simulink model "Crazyflie_NoLinealModel_EB_2020b"  (R2020b)
settings: Solver=FixedStepAuto  StartTime=0.0  StopTime=30  FixedStep=0.001  RelTol=1e-3
undefined symbols (not defined in the file): DiscIntNeverNeededParam, Dphi_s, Dphi_T, Dpsi_s, Dtheta_s, fm, MCO, Phi_s, Phi_T, phi_theta_limit, quad, Theta_s, U_q, V_q, we, X_q, XY_delta, XY_T, xyv_lim, Y_q, Yaw_delta, Yaw_q, Yaw_T, Z_delta, Z_s, Z_T
libraries: pid_lib x6, simulink x4
settings Model: Creator=Rafael  LastModifiedBy=FranciscoJose
settings DataIOCC: LimitDataPoints=on  SaveFormat=Array  SignalLoggingSaveFormat=ModelDataLogs  ReturnWorkspaceOutputs=off
settings OptimizationCC: ExpressionDepthLimit=2147483647  LifeSpan=inf
settings DebuggingCC: UnderspecifiedInitializationDetection=Classic  MergeDetectMultiDrivingBlocksExec=none  SolverPrmCheckMsg=warning  FcnCallInpInsideContextMsg=warning  AllowSymbolicDim=off  StateNameClashWarn=warning  SFUnexpectedBacktrackingDiag=warning  SFNoUnconditionalDefaultTransitionDiag=warning  SFExecutionAtInitializationDiag=none  ArithmeticOperatorsInVariantConditions=warning
settings HardwareCC: ProdBitPerPointer=32  ProdBitPerSizeT=32  ProdBitPerPtrDiffT=32  ProdLargestAtomicFloat=None  ProdIntDivRoundTo=Undefined  ProdEndianess=Unspecified  ProdWordSize=32  ProdHWDeviceType=32-bit Generic
settings ModelReferenceCC: PropagateSignalLabelsOutOfModel=off
settings SFSimCC: SimUseLocalCustomCode=off  CustomCodeUndefinedFunction=UseInterfaceOnly
settings RTWCC: RTWUseLocalCustomCode=off
settings CodeAppCC: StateflowObjectComments=on
settings GRTTargetCC: TargetLangStandard=C89/C90 (ANSI)
settings ConfigComp: CovMetricSettings=dw  CovSaveCumulativeToWorkspaceVar=on  CovSaveSingleToWorkspaceVar=on  CovExternalEMLEnable=off
settings SimscapeCC: SimscapeNormalizeSystem=off
settings ConfigurationSet: Description=SimMechanics 2G

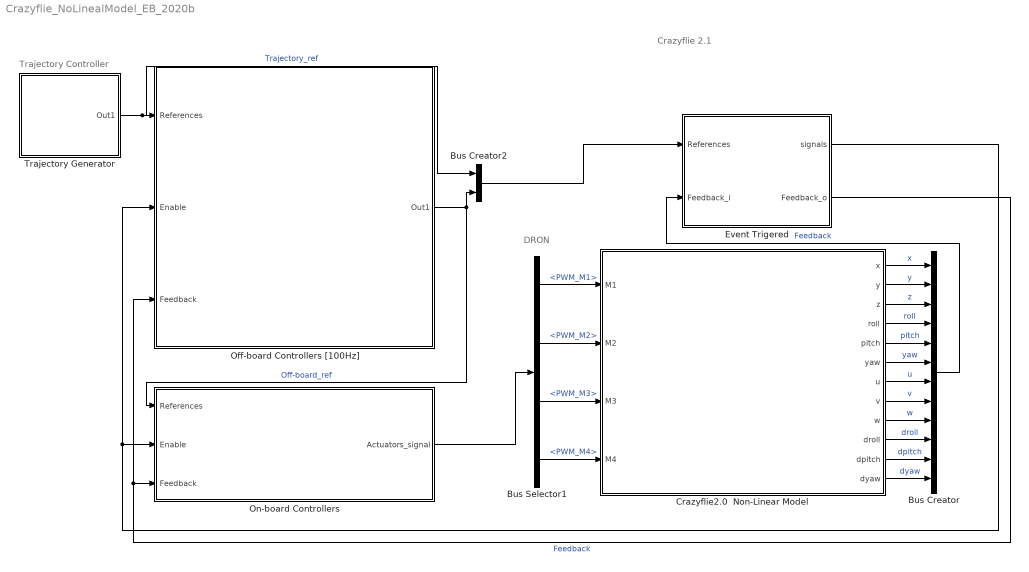
== system Crazyflie_NoLinealModel_EB_2020b ==
  note: DRON
  note: Trajectory Controller
  note: Crazyflie 2.1
  Bus Creator : BusCreator  Inputs=12
  Bus Creator2 : BusCreator  Inputs=2
  Bus Selector1 : BusSelector  OutputSignals=PWM_M1,PWM_M2,PWM_M3,PWM_M4
  Crazyflie2.0  Non-Linear Model : Subsystem
      mask Display: image('crazyflie_icon.png')
  Event Trigered : Subsystem
  Off-board Controllers [100Hz] : Subsystem
  On-board Controllers : Subsystem
  Trajectory Generator : Subsystem
  wires:
  Crazyflie2.0  Non-Linear Model/11(dpitch) -> Bus Creator/11  "dpitch"
  Crazyflie2.0  Non-Linear Model/3(z) -> Bus Creator/3  "z"
  Crazyflie2.0  Non-Linear Model/12(dyaw) -> Bus Creator/12  "dyaw"
  Crazyflie2.0  Non-Linear Model/4(roll) -> Bus Creator/4  "roll"
  Crazyflie2.0  Non-Linear Model/5(pitch) -> Bus Creator/5  "pitch"
  Crazyflie2.0  Non-Linear Model/6(yaw) -> Bus Creator/6  "yaw"
  Crazyflie2.0  Non-Linear Model/1(x) -> Bus Creator/1  "x"
  Crazyflie2.0  Non-Linear Model/2(y) -> Bus Creator/2  "y"
  Crazyflie2.0  Non-Linear Model/7(u) -> Bus Creator/7  "u"
  Crazyflie2.0  Non-Linear Model/8(v) -> Bus Creator/8  "v"
  Crazyflie2.0  Non-Linear Model/9(w) -> Bus Creator/9  "w"
  Crazyflie2.0  Non-Linear Model/10(droll) -> Bus Creator/10  "droll"
  Event Trigered/2(Feedback_o) -> Off-board Controllers [100Hz]/3(Feedback), On-board Controllers/3(Feedback)  "Feedback"
  Bus Selector1/1 -> Crazyflie2.0  Non-Linear Model/1(M1)  "<PWM_M1>"
  Bus Selector1/2 -> Crazyflie2.0  Non-Linear Model/2(M2)  "<PWM_M2>"
  Bus Selector1/3 -> Crazyflie2.0  Non-Linear Model/3(M3)  "<PWM_M3>"
  Bus Selector1/4 -> Crazyflie2.0  Non-Linear Model/4(M4)  "<PWM_M4>"
  Trajectory Generator/1(Out1) -> Bus Creator2/1, Off-board Controllers [100Hz]/1(References)  "Trajectory_ref"
  Bus Creator2/1 -> Event Trigered/1(References)
  Bus Creator/1 -> Event Trigered/2(Feedback_i)  "Feedback"
  Event Trigered/1(signals) -> Off-board Controllers [100Hz]/2(Enable), On-board Controllers/2(Enable)
  On-board Controllers/1(Actuators_signal) -> Bus Selector1/1
  Off-board Controllers [100Hz]/1(Out1) -> On-board Controllers/1(References), Bus Creator2/2  "Off-board_ref"

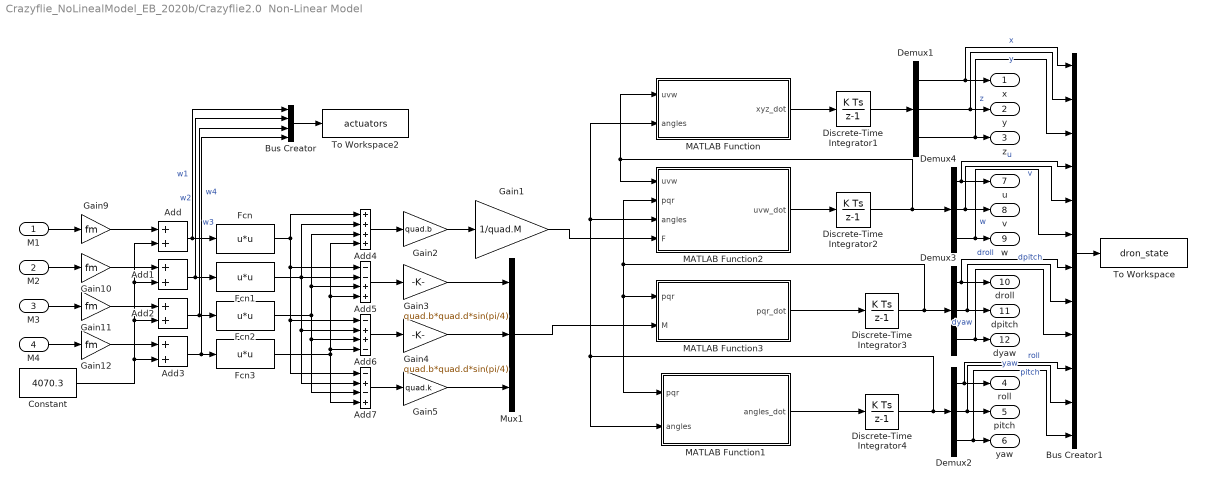
== system Crazyflie_NoLinealModel_EB_2020b/Crazyflie2.0  Non-Linear Model ==
  M1 : Inport
  M2 : Inport  Port=2
  M3 : Inport  Port=3
  M4 : Inport  Port=4
  Add{,1..3} (4 alike) : Sum
  Add4 : Sum  Inputs=++++
  Add5 : Sum  Inputs=--++
  Add6 : Sum  Inputs=-++-
  Add7 : Sum  Inputs=-+-+
  Bus Creator : BusCreator  Inputs=4
  Bus Creator1 : BusCreator  Inputs=12
  Constant : Constant  Value=4070.3
  Demux{1..4} (4 alike) : Demux  Outputs=3
  Discrete-Time Integrator{1..4} (4 alike) : DiscreteIntegrator  SampleTime=0.001  ICPrevOutput=DiscIntNeverNeededParam  ICPrevScaledInput=DiscIntNeverNeededParam
  Fcn{,1..3} (4 alike) : Fcn  Expr=u*u
  Gain1 : Gain  Gain=1/quad.M
  Gain{9..12} (4 alike) : Gain  Gain=fm
  Gain2 : Gain  Gain=quad.b
  Gain3 : Gain  Gain=quad.b*quad.d*sin(pi/4)
  Gain4 : Gain  Gain=quad.b*quad.d*sin(pi/4)
  Gain5 : Gain  Gain=quad.k
  MATLAB Function : MATLAB Function  TreatAsAtomicUnit=on
  MATLAB Function1 : MATLAB Function  TreatAsAtomicUnit=on
  MATLAB Function2 : MATLAB Function  TreatAsAtomicUnit=on
  MATLAB Function3 : MATLAB Function  TreatAsAtomicUnit=on
  Mux1 : Mux  Inputs=3
  To Workspace : ToWorkspace  VariableName=dron_state  SaveFormat=Timeseries  SampleTime=-1
  To Workspace2 : ToWorkspace  VariableName=actuators  SaveFormat=Timeseries  SampleTime=-1
  x : Outport
  y : Outport  Port=2
  z : Outport  Port=3
  roll : Outport  Port=4
  pitch : Outport  Port=5
  yaw : Outport  Port=6
  u : Outport  Port=7
  v : Outport  Port=8
  w : Outport  Port=9
  droll : Outport  Port=10
  dpitch : Outport  Port=11
  dyaw : Outport  Port=12
  wires:
  Demux1/1 -> Bus Creator1/1, x/1  "x"
  Demux1/2 -> Bus Creator1/2, y/1  "y"
  Demux2/1 -> Bus Creator1/10, roll/1  "roll"
  Demux2/2 -> Bus Creator1/11, pitch/1  "pitch"
  Demux2/3 -> Bus Creator1/12, yaw/1  "yaw"
  Demux4/1 -> Bus Creator1/4, u/1  "u"
  Demux4/2 -> Bus Creator1/5, v/1  "v"
  Demux4/3 -> Bus Creator1/6, w/1  "w"
  Demux3/1 -> Bus Creator1/7, droll/1  "droll"
  Demux3/2 -> Bus Creator1/8, dpitch/1  "dpitch"
  Demux3/3 -> Bus Creator1/9, dyaw/1  "dyaw"
  M1/1 -> Gain9/1
  M2/1 -> Gain10/1
  M3/1 -> Gain11/1
  M4/1 -> Gain12/1
  Add/1 -> Bus Creator/1, Fcn/1  "w1"
  Add1/1 -> Bus Creator/2, Fcn1/1  "w2"
  Add2/1 -> Bus Creator/3, Fcn2/1  "w3"
  Add3/1 -> Bus Creator/4, Fcn3/1  "w4"
  Gain9/1 -> Add/1
  Gain10/1 -> Add1/1
  Gain11/1 -> Add2/1
  Gain12/1 -> Add3/1
  Constant/1 -> Add3/2, Add/2, Add1/2, Add2/2
  Discrete-Time Integrator3/1 -> Demux3/1, MATLAB Function2/2(pqr), MATLAB Function1/1(pqr), MATLAB Function3/1(pqr)
  Discrete-Time Integrator2/1 -> MATLAB Function2/1(uvw), MATLAB Function/1(uvw), Demux4/1
  MATLAB Function3/1(pqr_dot) -> Discrete-Time Integrator3/1
  MATLAB Function1/1(angles_dot) -> Discrete-Time Integrator4/1
  Mux1/1 -> MATLAB Function3/2(M)
  Discrete-Time Integrator4/1 -> Demux2/1, MATLAB Function1/2(angles), MATLAB Function/2(angles), MATLAB Function2/3(angles)
  Discrete-Time Integrator1/1 -> Demux1/1
  MATLAB Function/1(xyz_dot) -> Discrete-Time Integrator1/1
  Gain4/1 -> Mux1/2
  Add6/1 -> Gain4/1
  Gain5/1 -> Mux1/3
  Gain3/1 -> Mux1/1
  Gain1/1 -> MATLAB Function2/4(F)
  Fcn2/1 -> Add4/3, Add5/3, Add7/3, Add6/3
  Add7/1 -> Gain5/1
  Fcn/1 -> Add4/1, Add7/1, Add6/1, Add5/1
  Add5/1 -> Gain3/1
  Fcn3/1 -> Add4/4, Add5/4, Add6/4, Add7/4
  Fcn1/1 -> Add4/2, Add7/2, Add6/2, Add5/2
  Gain2/1 -> Gain1/1
  Add4/1 -> Gain2/1
  MATLAB Function2/1(uvw_dot) -> Discrete-Time Integrator2/1
  Bus Creator/1 -> To Workspace2/1
  Bus Creator1/1 -> To Workspace/1
  Demux1/3 -> Bus Creator1/3, z/1  "z"

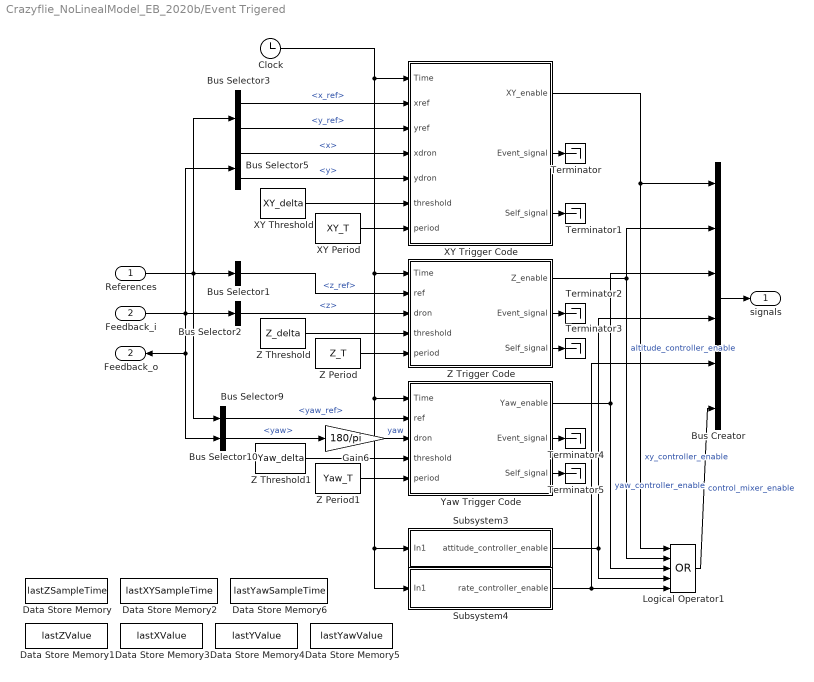
== system Crazyflie_NoLinealModel_EB_2020b/Event Trigered ==
  References : Inport
  Feedback_i : Inport  Port=2
  Bus Creator : BusCreator  Inputs=6
  Bus Selector1 : BusSelector  OutputSignals=Trajectory_ref.z_ref
  Bus Selector10 : BusSelector  OutputSignals=yaw
  Bus Selector2 : BusSelector  OutputSignals=z
  Bus Selector3 : BusSelector  OutputSignals=Trajectory_ref.x_ref,Trajectory_ref.y_ref
  Bus Selector5 : BusSelector  OutputSignals=x,y
  Bus Selector9 : BusSelector  OutputSignals=Trajectory_ref.yaw_ref
  Clock : Clock
  Data Store Memory : DataStoreMemory  DataStoreName=lastZSampleTime  InitialValue=0.0  ShowAdditionalParam=off  OutDataTypeStr=double
  Data Store Memory1 : DataStoreMemory  DataStoreName=lastZValue  InitialValue=0.0  ShowAdditionalParam=off  OutDataTypeStr=double
  Data Store Memory2 : DataStoreMemory  DataStoreName=lastXYSampleTime  InitialValue=0.0  ShowAdditionalParam=off  OutDataTypeStr=double
  Data Store Memory3 : DataStoreMemory  DataStoreName=lastXValue  InitialValue=0.0  ShowAdditionalParam=off  OutDataTypeStr=double
  Data Store Memory4 : DataStoreMemory  DataStoreName=lastYValue  InitialValue=0.0  ShowAdditionalParam=off  OutDataTypeStr=double
  Data Store Memory5 : DataStoreMemory  DataStoreName=lastYawValue  InitialValue=0.0  ShowAdditionalParam=off  OutDataTypeStr=double
  Data Store Memory6 : DataStoreMemory  DataStoreName=lastYawSampleTime  InitialValue=0.0  ShowAdditionalParam=off  OutDataTypeStr=double
  Gain6 : Gain  Gain=180/pi
  Logical Operator1 : Logic  Operator=OR  Inputs=5  AllPortsSameDT=off  OutDataTypeStr=boolean
  Subsystem3 : Subsystem
  Subsystem4 : Subsystem
  Terminator{,1..5} (6 alike) : Terminator
  XY Period : Constant  Value=XY_T
  XY Threshold : Constant  Value=XY_delta
  XY Trigger Code : MATLAB Function  TreatAsAtomicUnit=on
  Yaw Trigger Code : MATLAB Function  TreatAsAtomicUnit=on
  Z Period : Constant  Value=Z_T
  Z Period1 : Constant  Value=Yaw_T
  Z Threshold : Constant  Value=Z_delta
  Z Threshold1 : Constant  Value=Yaw_delta
  Z Trigger Code : MATLAB Function  TreatAsAtomicUnit=on
  signals : Outport
  Feedback_o : Outport  Port=2
  wires:
  References/1 -> Bus Selector9/1, Bus Selector1/1, Bus Selector3/1
  Bus Selector9/1 -> Yaw Trigger Code/2(ref)  "<yaw_ref>"
  Bus Selector10/1 -> Gain6/1  "<yaw>"
  Bus Creator/1 -> signals/1
  Gain6/1 -> Yaw Trigger Code/3(dron)  "yaw"
  Logical Operator1/1 -> Bus Creator/6  "control_mixer_enable"
  Z Trigger Code/1(Z_enable) -> Logical Operator1/2, Bus Creator/2  "altitude_controller_enable"
  XY Trigger Code/1(XY_enable) -> Logical Operator1/1, Bus Creator/1  "xy_controller_enable"
  Yaw Trigger Code/1(Yaw_enable) -> Logical Operator1/3, Bus Creator/3  "yaw_controller_enable"
  Subsystem3/1(attitude_controller_enable) -> Bus Creator/4, Logical Operator1/4
  Clock/1 -> Subsystem4/1(In1), Subsystem3/1(In1), Yaw Trigger Code/1(Time), Z Trigger Code/1(Time), XY Trigger Code/1(Time)
  Subsystem4/1(rate_controller_enable) -> Logical Operator1/5, Bus Creator/5
  Z Threshold/1 -> Z Trigger Code/4(threshold)
  Z Period/1 -> Z Trigger Code/5(period)
  Bus Selector1/1 -> Z Trigger Code/2(ref)  "<z_ref>"
  Bus Selector2/1 -> Z Trigger Code/3(dron)  "<z>"
  Bus Selector3/1 -> XY Trigger Code/2(xref)  "<x_ref>"
  Bus Selector3/2 -> XY Trigger Code/3(yref)  "<y_ref>"
  Feedback_i/1 -> Bus Selector2/1, Bus Selector5/1, Bus Selector10/1, Feedback_o/1
  Bus Selector5/1 -> XY Trigger Code/4(xdron)  "<x>"
  Bus Selector5/2 -> XY Trigger Code/5(ydron)  "<y>"
  XY Threshold/1 -> XY Trigger Code/6(threshold)
  XY Period/1 -> XY Trigger Code/7(period)
  XY Trigger Code/2(Event_signal) -> Terminator/1
  XY Trigger Code/3(Self_signal) -> Terminator1/1
  Z Threshold1/1 -> Yaw Trigger Code/4(threshold)
  Z Period1/1 -> Yaw Trigger Code/5(period)
  Yaw Trigger Code/2(Event_signal) -> Terminator4/1
  Yaw Trigger Code/3(Self_signal) -> Terminator5/1
  Z Trigger Code/2(Event_signal) -> Terminator2/1
  Z Trigger Code/3(Self_signal) -> Terminator3/1

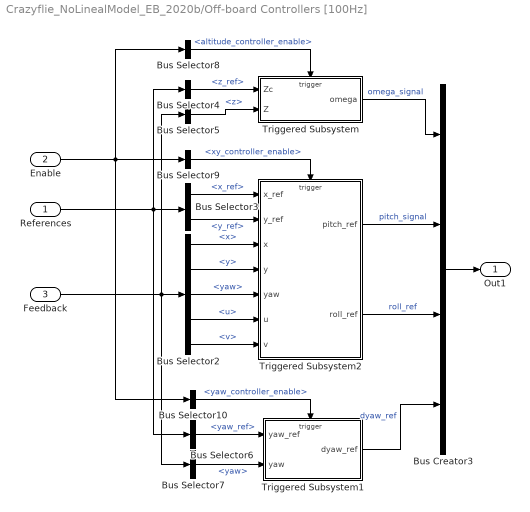
== system Crazyflie_NoLinealModel_EB_2020b/Off-board Controllers [100Hz] ==
  References : Inport
  Enable : Inport  Port=2
  Feedback : Inport  Port=3
  Bus Creator3 : BusCreator  Inputs=4
  Bus Selector10 : BusSelector  OutputSignals=yaw_controller_enable
  Bus Selector2 : BusSelector  OutputSignals=x,y,yaw,u,v
  Bus Selector3 : BusSelector  OutputSignals=x_ref,y_ref
  Bus Selector4 : BusSelector  OutputSignals=z_ref
  Bus Selector5 : BusSelector  OutputSignals=z
  Bus Selector6 : BusSelector  OutputSignals=yaw_ref
  Bus Selector7 : BusSelector  OutputSignals=yaw
  Bus Selector8 : BusSelector  OutputSignals=altitude_controller_enable
  Bus Selector9 : BusSelector  OutputSignals=xy_controller_enable
  Triggered Subsystem : Subsystem  TreatAsAtomicUnit=on
  Triggered Subsystem1 : Subsystem  TreatAsAtomicUnit=on
  Triggered Subsystem2 : Subsystem  TreatAsAtomicUnit=on
  Out1 : Outport
  wires:
  Bus Selector2/3 -> Triggered Subsystem2/5(yaw)  "<yaw>"
  Bus Selector6/1 -> Triggered Subsystem1/1(yaw_ref)  "<yaw_ref>"
  Bus Selector2/5 -> Triggered Subsystem2/7(v)  "<v>"
  References/1 -> Bus Selector4/1, Bus Selector3/1, Bus Selector6/1
  Triggered Subsystem2/1(pitch_ref) -> Bus Creator3/2  "pitch_signal"
  Enable/1 -> Bus Selector10/1, Bus Selector8/1, Bus Selector9/1
  Feedback/1 -> Bus Selector7/1, Bus Selector5/1, Bus Selector2/1
  Bus Selector2/1 -> Triggered Subsystem2/3(x)  "<x>"
  Bus Selector7/1 -> Triggered Subsystem1/2(yaw)  "<yaw>"
  Bus Selector2/4 -> Triggered Subsystem2/6(u)  "<u>"
  Bus Selector4/1 -> Triggered Subsystem/1(Zc)  "<z_ref>"
  Bus Selector3/1 -> Triggered Subsystem2/1(x_ref)  "<x_ref>"
  Bus Selector3/2 -> Triggered Subsystem2/2(y_ref)  "<y_ref>"
  Bus Selector2/2 -> Triggered Subsystem2/4(y)  "<y>"
  Triggered Subsystem2/2(roll_ref) -> Bus Creator3/3  "roll_ref"
  Bus Selector5/1 -> Triggered Subsystem/2(Z)  "<z>"
  Triggered Subsystem1/1(dyaw_ref) -> Bus Creator3/4  "dyaw_ref"
  Bus Selector9/1 -> Triggered Subsystem2/Trigger  "<xy_controller_enable>"
  Bus Selector10/1 -> Triggered Subsystem1/Trigger  "<yaw_controller_enable>"
  Bus Selector8/1 -> Triggered Subsystem/Trigger  "<altitude_controller_enable>"
  Bus Creator3/1 -> Out1/1
  Triggered Subsystem/1(omega) -> Bus Creator3/1  "omega_signal"

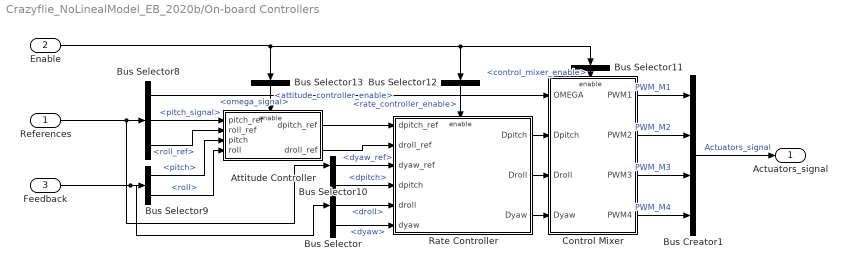
== system Crazyflie_NoLinealModel_EB_2020b/On-board Controllers ==
  References : Inport
  Enable : Inport  Port=2
  Feedback : Inport  Port=3
  Attitude Controller : Subsystem  TreatAsAtomicUnit=on
  Bus Creator1 : BusCreator  Inputs=4
  Bus Selector : BusSelector  OutputSignals=dpitch,droll,dyaw
  Bus Selector10 : BusSelector  OutputSignals=dyaw_ref
  Bus Selector11 : BusSelector  OutputSignals=control_mixer_enable
  Bus Selector12 : BusSelector  OutputSignals=rate_controller_enable
  Bus Selector13 : BusSelector  OutputSignals=attitude_controller_enable
  Bus Selector8 : BusSelector  OutputSignals=omega_signal,pitch_signal,roll_ref
  Bus Selector9 : BusSelector  OutputSignals=pitch,roll
  Control Mixer : Subsystem  TreatAsAtomicUnit=on
  Rate Controller : Subsystem  TreatAsAtomicUnit=on
  Actuators_signal : Outport
  wires:
  Bus Creator1/1 -> Actuators_signal/1  "Actuators_signal"
  Bus Selector/2 -> Rate Controller/5(droll)  "<droll>"
  Control Mixer/3(PWM3) -> Bus Creator1/3  "PWM_M3"
  Rate Controller/3(Dyaw) -> Control Mixer/4(Dyaw)
  Enable/1 -> Bus Selector11/1, Bus Selector12/1, Bus Selector13/1
  Bus Selector8/2 -> Attitude Controller/1(pitch_ref)  "<pitch_signal>"
  Bus Selector8/3 -> Attitude Controller/2(roll_ref)  "<roll_ref>"
  References/1 -> Bus Selector8/1, Bus Selector10/1
  Bus Selector12/1 -> Rate Controller/Enable  "<rate_controller_enable>"
  Attitude Controller/2(droll_ref) -> Rate Controller/2(droll_ref)
  Bus Selector10/1 -> Rate Controller/3(dyaw_ref)  "<dyaw_ref>"
  Bus Selector/1 -> Rate Controller/4(dpitch)  "<dpitch>"
  Bus Selector/3 -> Rate Controller/6(dyaw)  "<dyaw>"
  Feedback/1 -> Bus Selector/1, Bus Selector9/1
  Control Mixer/4(PWM4) -> Bus Creator1/4  "PWM_M4"
  Attitude Controller/1(dpitch_ref) -> Rate Controller/1(dpitch_ref)
  Rate Controller/1(Dpitch) -> Control Mixer/2(Dpitch)
  Rate Controller/2(Droll) -> Control Mixer/3(Droll)
  Bus Selector8/1 -> Control Mixer/1(OMEGA)  "<omega_signal>"
  Control Mixer/2(PWM2) -> Bus Creator1/2  "PWM_M2"
  Control Mixer/1(PWM1) -> Bus Creator1/1  "PWM_M1"
  Bus Selector9/2 -> Attitude Controller/4(roll)  "<roll>"
  Bus Selector9/1 -> Attitude Controller/3(pitch)  "<pitch>"
  Bus Selector11/1 -> Control Mixer/Enable  "<control_mixer_enable>"
  Bus Selector13/1 -> Attitude Controller/Enable  "<attitude_controller_enable>"

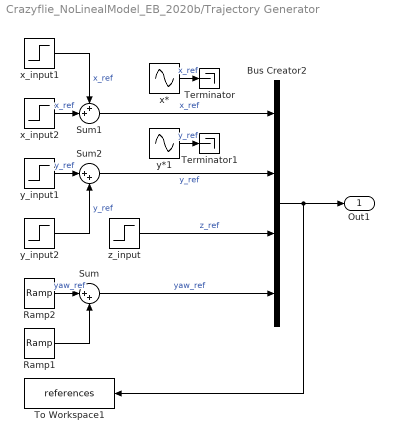
== system Crazyflie_NoLinealModel_EB_2020b/Trajectory Generator ==
  Bus Creator2 : BusCreator  Inputs=4
  Ramp1 : simulink/Sources/Ramp  slope=-pi/3  start=10  InitialOutput=0
  Ramp2 : simulink/Sources/Ramp  slope=pi/3  start=0  InitialOutput=0
  Sum : Sum  Inputs=|++
  Sum1 : Sum  Inputs=++|
  Sum2 : Sum  Inputs=|++
  Terminator : Terminator
  Terminator1 : Terminator
  To Workspace1 : ToWorkspace  VariableName=references  SaveFormat=Timeseries  SampleTime=-1
  x* : Sin  Amplitude=0.8  Frequency=2*pi*0.085  Phase=0-0.1  SampleTime=0
  x_input1 : Step  Time=6  SampleTime=0
  x_input2 : Step  Time=18  After=-1  SampleTime=0
  y*1 : Sin  Amplitude=0.8  Frequency=2*pi*0.085  Phase=pi/2-0.1  SampleTime=0
  y_input1 : Step  Time=12  SampleTime=0
  y_input2 : Step  Time=24  After=-1  SampleTime=0
  z_input : Step  Time=0  SampleTime=0
  Out1 : Outport
  wires:
  z_input/1 -> Bus Creator2/3  "z_ref"
  Sum1/1 -> Bus Creator2/1  "x_ref"
  Ramp1/1 -> Sum/2
  Sum2/1 -> Bus Creator2/2  "y_ref"
  Bus Creator2/1 -> To Workspace1/1, Out1/1
  Sum/1 -> Bus Creator2/4  "yaw_ref"
  Ramp2/1 -> Sum/1  "yaw_ref"
  x_input2/1 -> Sum1/2  "x_ref"
  x_input1/1 -> Sum1/1  "x_ref"
  y_input1/1 -> Sum2/1  "y_ref"
  y_input2/1 -> Sum2/2  "y_ref"
  x*/1 -> Terminator/1  "x_ref"
  y*1/1 -> Terminator1/1  "y_ref"

== system Crazyflie_NoLinealModel_EB_2020b/Event Trigered/Subsystem3 ==
  In1 : Inport
  Compare To Constant4 : simulink/Logic and Bit Operations/Compare To Constant  relop=>=  const=Phi_T  OutDataTypeStr=boolean
  If Action Subsystem4 : Subsystem  TreatAsAtomicUnit=on
  Memory4 : Memory
  Sum8 : Sum  Inputs=|+-
  attitude_controller_enable : Outport
  wires:
  In1/1 -> Sum8/1, If Action Subsystem4/1(In2)
  If Action Subsystem4/1(Out2) -> Memory4/1
  Compare To Constant4/1 -> attitude_controller_enable/1, If Action Subsystem4/Enable  "attitude_controller_enable"
  Memory4/1 -> Sum8/2
  Sum8/1 -> Compare To Constant4/1

== system Crazyflie_NoLinealModel_EB_2020b/Event Trigered/Subsystem4 ==
  In1 : Inport
  Compare To Constant4 : simulink/Logic and Bit Operations/Compare To Constant  relop=>=  const=Dphi_T  OutDataTypeStr=boolean
  If Action Subsystem4 : Subsystem  TreatAsAtomicUnit=on
  Memory4 : Memory
  Sum8 : Sum  Inputs=|+-
  rate_controller_enable : Outport
  wires:
  In1/1 -> Sum8/1, If Action Subsystem4/1(In2)
  Sum8/1 -> Compare To Constant4/1
  If Action Subsystem4/1(Out2) -> Memory4/1
  Compare To Constant4/1 -> rate_controller_enable/1, If Action Subsystem4/Enable  "rate_controller_enable"
  Memory4/1 -> Sum8/2

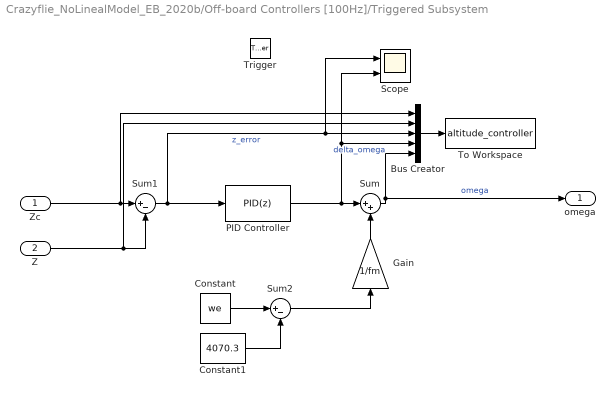
== system Crazyflie_NoLinealModel_EB_2020b/Off-board Controllers [100Hz]/Triggered Subsystem ==
  Zc : Inport
  Z : Inport  Port=2
  Trigger : TriggerPort  VariantControl=Variant
  Bus Creator : BusCreator  Inputs=5
  Constant : Constant  Value=we
  Constant1 : Constant  Value=4070.3
  Gain : Gain  Gain=1/fm
  PID Controller : pid_lib/PID Controller  Controller=PID  Form=Parallel  TimeDomain=Discrete-time  UseExternalTs=off  SampleTime=-1  IntegratorMethod=Forward Euler  FilterMethod=Forward Euler  ControllerParametersSource=internal  P=Z_s(1)  I=Z_s(2)  D=Z_s(3)  UseFilter=on  N=100  TunerSelectOption=Transfer Function Based (PID Tuner App)  InitialConditionSource=internal  InitialConditionForIntegrator=0  InitialConditionForFilter=0  DifferentiatorICPrevScaledInput=0  ExternalReset=none  TrackingMode=off  Kt=1  LimitOutput=on  SatLimitsSource=internal  UpperSaturationLimit=15000  LowerSaturationLimit=-20000  LinearizeAsGain=on  AntiWindupMode=none  Kb=1/sqrt(0.75)  POutMin=[]  POutMax=[]  IOutMin=[]  IOutMax=[]  DOutMin=[]  DOutMax=[]  NOutMin=[]  NOutMax=[]  SumOutMin=[]  SumOutMax=[]  SaturationOutMin=[]  SaturationOutMax=[]  PParamMin=[]  PParamMax=[]  IParamMin=[]  IParamMax=[]  DParamMin=[]  DParamMax=[]  NParamMin=[]  NParamMax=[]  KbParamMin=[]  KbParamMax=[]  KtParamMin=[]  KtParamMax=[]  KbOutMin=[]  KbOutMax=[]  KtOutMin=[]  KtOutMax=[]  IntegratorOutMin=[]  IntegratorOutMax=[]  FilterOutMin=[]  FilterOutMax=[]  SumI1OutMin=[]  SumI1OutMax=[]  SumI2OutMin=[]  SumI2OutMax=[]  SumI3OutMin=[]  SumI3OutMax=[]  SumI4OutMin=[]  SumI4OutMax=[]  SumDOutMin=[]  SumDOutMax=[]  DifferentiatorOutMin=[]  DifferentiatorOutMax=[]  FilterDiffOutCoefMin=[]  FilterDiffOutCoefMax=[]  ReciprocalOutMin=[]  ReciprocalOutMax=[]  SumDenOutMin=[]  SumDenOutMax=[]  SumNumOutMin=[]  SumNumOutMax=[]  DivideOutMin=[]  DivideOutMax=[]  UdiffTsProdOutMin=[]  UdiffTsProdOutMax=[]  NTsProdOutMin=[]  NTsProdOutMax=[]  UintegralTsProdOutMin=[]  UintegralTsProdOutMax=[]  UngainTsProdOutMin=[]  UngainTsProdOutMax=[]  IntegratorContinuousStateAttributes=''  IntegratorStateMustResolveToSignalObject=off  IntegratorRTWStateStorageClass=Auto  FilterContinuousStateAttributes=''  FilterStateMustResolveToSignalObject=off  FilterRTWStateStorageClass=Auto  ParallelPVariant=InternalParameters  IdealPVariant=Disabled  IVariant=InternalParameters  DVariant=InternalParameters  IntegratorVariant=Discrete  SatVariant=Enabled  AWVariant=Passthrough  PCopyVariant=Disabled  TRVariant=Disabled  FdbkBlocksVariant=Forward  IdealPFdbkVariant=Disabled  SatFdbkVariant=Disabled  DerivativeFilterVariant=ForwardEulerFilter  NVariant=InternalParameters  NCopyVariant=Disabled  FilterICVariant=InternalICsFilter  IntegratorICVariant=InternalICs  ExternalResetVariant=Disabled  TRSumVariant=Passthrough  SumFdbkVariant=Disabled  SumVariant=Sum_PID  TsampFilterVariant=InternalTs  TsampNgainVariant=Passthrough  TsampIntegralVariant=Passthrough  ExternalSaturationOutDataTypeStr=Inherit: Same as second input
  Scope : Scope  NumInputPorts=2
  Sum : Sum  Inputs=|++
  Sum1 : Sum  Inputs=|+-
  Sum2 : Sum  Inputs=|+-
  To Workspace : ToWorkspace  VariableName=altitude_controller  SaveFormat=Timeseries  SampleTime=-1
  omega : Outport
  wires:
  Gain/1 -> Sum/2
  Constant/1 -> Sum2/1
  Bus Creator/1 -> To Workspace/1
  Constant1/1 -> Sum2/2
  Zc/1 -> Bus Creator/1, Sum1/1
  Sum/1 -> Bus Creator/5, omega/1  "omega"
  Sum2/1 -> Gain/1
  Sum1/1 -> PID Controller/1, Scope/1, Bus Creator/3  "z_error"
  Z/1 -> Bus Creator/2, Sum1/2
  PID Controller/1 -> Scope/2, Bus Creator/4, Sum/1  "delta_omega"

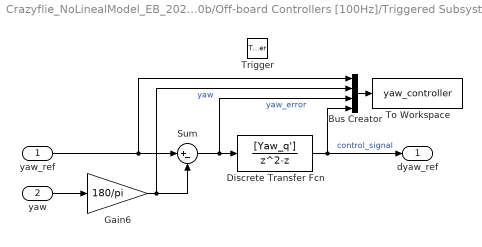
== system Crazyflie_NoLinealModel_EB_2020b/Off-board Controllers [100Hz]/Triggered Subsystem1 ==
  yaw_ref : Inport
  yaw : Inport  Port=2
  Trigger : TriggerPort  VariantControl=Variant
  Bus Creator : BusCreator  Inputs=4
  Discrete Transfer Fcn : DiscreteTransferFcn  Numerator=[Yaw_q']  Denominator=[1 -1 0]
  Gain6 : Gain  Gain=180/pi
  Sum : Sum  Inputs=|+-
  To Workspace : ToWorkspace  VariableName=yaw_controller  SaveFormat=Timeseries  SampleTime=-1
  dyaw_ref : Outport
  wires:
  Sum/1 -> Discrete Transfer Fcn/1, Bus Creator/3  "yaw_error"
  Discrete Transfer Fcn/1 -> Bus Creator/4, dyaw_ref/1  "control_signal"
  Gain6/1 -> Bus Creator/2, Sum/2  "yaw"
  yaw/1 -> Gain6/1
  yaw_ref/1 -> Bus Creator/1, Sum/1
  Bus Creator/1 -> To Workspace/1

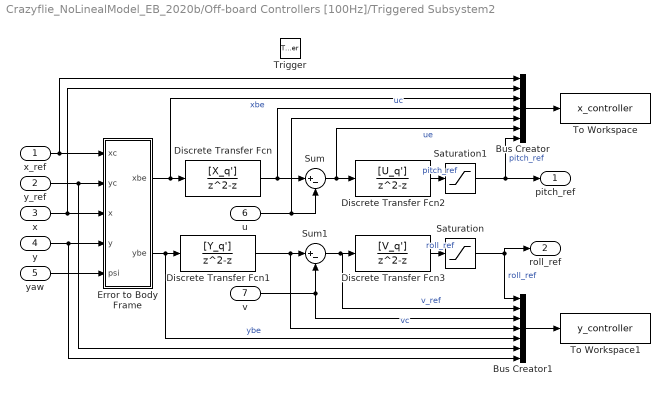
== system Crazyflie_NoLinealModel_EB_2020b/Off-board Controllers [100Hz]/Triggered Subsystem2 ==
  x_ref : Inport
  y_ref : Inport  Port=2
  x : Inport  Port=3
  y : Inport  Port=4
  yaw : Inport  Port=5
  u : Inport  Port=6
  v : Inport  Port=7
  Trigger : TriggerPort  VariantControl=Variant
  Bus Creator : BusCreator  Inputs=7
  Bus Creator1 : BusCreator  Inputs=7
  Discrete Transfer Fcn : DiscreteTransferFcn  Numerator=[X_q']  Denominator=[1 -1 0]
  Discrete Transfer Fcn1 : DiscreteTransferFcn  Numerator=[Y_q']  Denominator=[1 -1 0]
  Discrete Transfer Fcn2 : DiscreteTransferFcn  Numerator=[U_q']  Denominator=[1 -1 0]
  Discrete Transfer Fcn3 : DiscreteTransferFcn  Numerator=[V_q']  Denominator=[1 -1 0]
  Error to Body Frame : MATLAB Function  TreatAsAtomicUnit=on
  Saturation : Saturate  UpperLimit=xyv_lim  LowerLimit=-xyv_lim
  Saturation1 : Saturate  UpperLimit=xyv_lim  LowerLimit=-xyv_lim
  Sum : Sum  Inputs=|+-
  Sum1 : Sum  Inputs=|+-
  To Workspace : ToWorkspace  VariableName=x_controller  SaveFormat=Timeseries  SampleTime=-1
  To Workspace1 : ToWorkspace  VariableName=y_controller  SaveFormat=Timeseries  SampleTime=-1
  pitch_ref : Outport
  roll_ref : Outport  Port=2
  wires:
  yaw/1 -> Error to Body Frame/5(psi)
  Discrete Transfer Fcn1/1 -> Bus Creator1/4, Sum1/1  "vc"
  Bus Creator1/1 -> To Workspace1/1
  v/1 -> Sum1/2, Bus Creator1/3
  Error to Body Frame/2(ybe) -> Bus Creator1/5, Discrete Transfer Fcn1/1  "ybe"
  y_ref/1 -> Bus Creator1/6, Error to Body Frame/2(yc)
  Bus Creator/1 -> To Workspace/1
  Error to Body Frame/1(xbe) -> Bus Creator/3, Discrete Transfer Fcn/1  "xbe"
  u/1 -> Bus Creator/5, Sum/2
  Saturation1/1 -> pitch_ref/1, Bus Creator/7  "pitch_ref"
  Sum/1 -> Discrete Transfer Fcn2/1, Bus Creator/6  "ue"
  y/1 -> Bus Creator1/7, Error to Body Frame/4(y)
  Discrete Transfer Fcn/1 -> Bus Creator/4, Sum/1  "uc"
  Saturation/1 -> Bus Creator1/1, roll_ref/1  "roll_ref"
  x_ref/1 -> Bus Creator/1, Error to Body Frame/1(xc)
  x/1 -> Bus Creator/2, Error to Body Frame/3(x)
  Sum1/1 -> Bus Creator1/2, Discrete Transfer Fcn3/1  "v_ref"
  Discrete Transfer Fcn2/1 -> Saturation1/1  "pitch_ref"
  Discrete Transfer Fcn3/1 -> Saturation/1  "roll_ref"

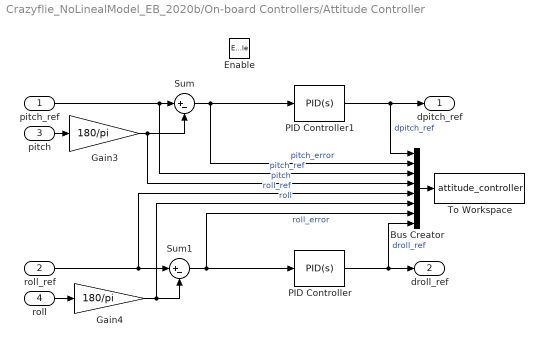
== system Crazyflie_NoLinealModel_EB_2020b/On-board Controllers/Attitude Controller ==
  pitch_ref : Inport
  roll_ref : Inport  Port=2
  pitch : Inport  Port=3
  roll : Inport  Port=4
  Enable : EnablePort
  Bus Creator : BusCreator  Inputs=8
  Gain3 : Gain  Gain=180/pi
  Gain4 : Gain  Gain=180/pi
  PID Controller : pid_lib/PID Controller  Controller=PID  Form=Parallel  TimeDomain=Continuous-time  UseExternalTs=off  SampleTime=-1  IntegratorMethod=Forward Euler  FilterMethod=Forward Euler  ControllerParametersSource=internal  P=Theta_s(1)  I=Theta_s(2)  D=Theta_s(3)  UseFilter=on  N=100  TunerSelectOption=Transfer Function Based (PID Tuner App)  InitialConditionSource=internal  InitialConditionForIntegrator=0  InitialConditionForFilter=0  DifferentiatorICPrevScaledInput=0  ExternalReset=none  TrackingMode=off  Kt=1  LimitOutput=on  SatLimitsSource=internal  UpperSaturationLimit=phi_theta_limit  LowerSaturationLimit=-phi_theta_limit  LinearizeAsGain=on  AntiWindupMode=back-calculation  Kb=1/sqrt(Theta_s(2))  POutMin=[]  POutMax=[]  IOutMin=[]  IOutMax=[]  DOutMin=[]  DOutMax=[]  NOutMin=[]  NOutMax=[]  SumOutMin=[]  SumOutMax=[]  SaturationOutMin=[]  SaturationOutMax=[]  PParamMin=[]  PParamMax=[]  IParamMin=[]  IParamMax=[]  DParamMin=[]  DParamMax=[]  NParamMin=[]  NParamMax=[]  KbParamMin=[]  KbParamMax=[]  KtParamMin=[]  KtParamMax=[]  KbOutMin=[]  KbOutMax=[]  KtOutMin=[]  KtOutMax=[]  IntegratorOutMin=[]  IntegratorOutMax=[]  FilterOutMin=[]  FilterOutMax=[]  SumI1OutMin=[]  SumI1OutMax=[]  SumI2OutMin=[]  SumI2OutMax=[]  SumI3OutMin=[]  SumI3OutMax=[]  SumI4OutMin=[]  SumI4OutMax=[]  SumDOutMin=[]  SumDOutMax=[]  DifferentiatorOutMin=[]  DifferentiatorOutMax=[]  FilterDiffOutCoefMin=[]  FilterDiffOutCoefMax=[]  ReciprocalOutMin=[]  ReciprocalOutMax=[]  SumDenOutMin=[]  SumDenOutMax=[]  SumNumOutMin=[]  SumNumOutMax=[]  DivideOutMin=[]  DivideOutMax=[]  UdiffTsProdOutMin=[]  UdiffTsProdOutMax=[]  NTsProdOutMin=[]  NTsProdOutMax=[]  UintegralTsProdOutMin=[]  UintegralTsProdOutMax=[]  UngainTsProdOutMin=[]  UngainTsProdOutMax=[]  IntegratorContinuousStateAttributes=''  IntegratorStateMustResolveToSignalObject=off  IntegratorRTWStateStorageClass=Auto  FilterContinuousStateAttributes=''  FilterStateMustResolveToSignalObject=off  FilterRTWStateStorageClass=Auto  ParallelPVariant=InternalParameters  IdealPVariant=Disabled  IVariant=InternalParameters  DVariant=InternalParameters  IntegratorVariant=Continuous  SatVariant=Enabled  AWVariant=BackCalculation  PCopyVariant=Disabled  TRVariant=Disabled  FdbkBlocksVariant=Forward  IdealPFdbkVariant=Disabled  SatFdbkVariant=Disabled  DerivativeFilterVariant=ContFilter  NVariant=InternalParameters  NCopyVariant=Disabled  FilterICVariant=InternalICsFilter  IntegratorICVariant=InternalICs  ExternalResetVariant=Disabled  TRSumVariant=Passthrough  SumFdbkVariant=Disabled  SumVariant=Sum_PID  TsampFilterVariant=InternalTs  TsampNgainVariant=Passthrough  TsampIntegralVariant=Passthrough  ExternalSaturationOutDataTypeStr=Inherit: Same as second input
  PID Controller1 : pid_lib/PID Controller  Controller=PID  Form=Parallel  TimeDomain=Continuous-time  UseExternalTs=off  SampleTime=-1  IntegratorMethod=Forward Euler  FilterMethod=Forward Euler  ControllerParametersSource=internal  P=Phi_s(1)  I=Phi_s(2)  D=Phi_s(3)  UseFilter=on  N=100  TunerSelectOption=Transfer Function Based (PID Tuner App)  InitialConditionSource=internal  InitialConditionForIntegrator=0  InitialConditionForFilter=0  DifferentiatorICPrevScaledInput=0  ExternalReset=none  TrackingMode=off  Kt=1  LimitOutput=on  SatLimitsSource=internal  UpperSaturationLimit=phi_theta_limit  LowerSaturationLimit=-phi_theta_limit  LinearizeAsGain=on  AntiWindupMode=back-calculation  Kb=1/sqrt(Phi_s(2))  POutMin=[]  POutMax=[]  IOutMin=[]  IOutMax=[]  DOutMin=[]  DOutMax=[]  NOutMin=[]  NOutMax=[]  SumOutMin=[]  SumOutMax=[]  SaturationOutMin=[]  SaturationOutMax=[]  PParamMin=[]  PParamMax=[]  IParamMin=[]  IParamMax=[]  DParamMin=[]  DParamMax=[]  NParamMin=[]  NParamMax=[]  KbParamMin=[]  KbParamMax=[]  KtParamMin=[]  KtParamMax=[]  KbOutMin=[]  KbOutMax=[]  KtOutMin=[]  KtOutMax=[]  IntegratorOutMin=[]  IntegratorOutMax=[]  FilterOutMin=[]  FilterOutMax=[]  SumI1OutMin=[]  SumI1OutMax=[]  SumI2OutMin=[]  SumI2OutMax=[]  SumI3OutMin=[]  SumI3OutMax=[]  SumI4OutMin=[]  SumI4OutMax=[]  SumDOutMin=[]  SumDOutMax=[]  DifferentiatorOutMin=[]  DifferentiatorOutMax=[]  FilterDiffOutCoefMin=[]  FilterDiffOutCoefMax=[]  ReciprocalOutMin=[]  ReciprocalOutMax=[]  SumDenOutMin=[]  SumDenOutMax=[]  SumNumOutMin=[]  SumNumOutMax=[]  DivideOutMin=[]  DivideOutMax=[]  UdiffTsProdOutMin=[]  UdiffTsProdOutMax=[]  NTsProdOutMin=[]  NTsProdOutMax=[]  UintegralTsProdOutMin=[]  UintegralTsProdOutMax=[]  UngainTsProdOutMin=[]  UngainTsProdOutMax=[]  IntegratorContinuousStateAttributes=''  IntegratorStateMustResolveToSignalObject=off  IntegratorRTWStateStorageClass=Auto  FilterContinuousStateAttributes=''  FilterStateMustResolveToSignalObject=off  FilterRTWStateStorageClass=Auto  ParallelPVariant=InternalParameters  IdealPVariant=Disabled  IVariant=InternalParameters  DVariant=InternalParameters  IntegratorVariant=Continuous  SatVariant=Enabled  AWVariant=BackCalculation  PCopyVariant=Disabled  TRVariant=Disabled  FdbkBlocksVariant=Forward  IdealPFdbkVariant=Disabled  SatFdbkVariant=Disabled  DerivativeFilterVariant=ContFilter  NVariant=InternalParameters  NCopyVariant=Disabled  FilterICVariant=InternalICsFilter  IntegratorICVariant=InternalICs  ExternalResetVariant=Disabled  TRSumVariant=Passthrough  SumFdbkVariant=Disabled  SumVariant=Sum_PID  TsampFilterVariant=InternalTs  TsampNgainVariant=Passthrough  TsampIntegralVariant=Passthrough  ExternalSaturationOutDataTypeStr=Inherit: Same as second input
  Sum : Sum  Inputs=|+-
  Sum1 : Sum  Inputs=|+-
  To Workspace : ToWorkspace  VariableName=attitude_controller  SaveFormat=Timeseries  SampleTime=-1
  dpitch_ref : Outport
  droll_ref : Outport  Port=2
  wires:
  pitch_ref/1 -> Bus Creator/3, Sum/1  "pitch_ref"
  Gain4/1 -> Bus Creator/6, Sum1/2  "roll"
  Sum/1 -> PID Controller1/1, Bus Creator/2  "pitch_error"
  roll_ref/1 -> Bus Creator/5, Sum1/1  "roll_ref"
  roll/1 -> Gain4/1
  Gain3/1 -> Bus Creator/4, Sum/2  "pitch"
  pitch/1 -> Gain3/1
  PID Controller1/1 -> Bus Creator/1, dpitch_ref/1  "dpitch_ref"
  Bus Creator/1 -> To Workspace/1
  PID Controller/1 -> Bus Creator/8, droll_ref/1  "droll_ref"
  Sum1/1 -> PID Controller/1, Bus Creator/7  "roll_error"

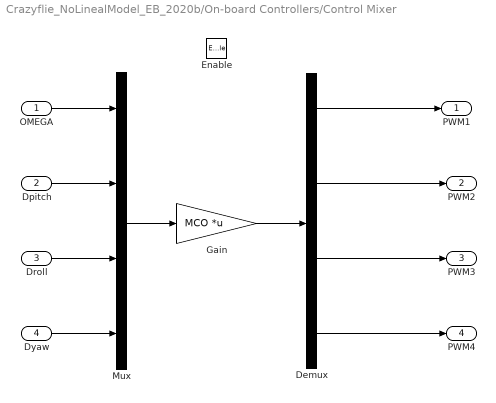
== system Crazyflie_NoLinealModel_EB_2020b/On-board Controllers/Control Mixer ==
  OMEGA : Inport
  Dpitch : Inport  Port=2
  Droll : Inport  Port=3
  Dyaw : Inport  Port=4
  Enable : EnablePort
  Demux : Demux
  Gain : Gain  Gain=MCO  Multiplication=Matrix(K*u) (u vector)
  Mux : Mux
  PWM1 : Outport
  PWM2 : Outport  Port=2
  PWM3 : Outport  Port=3
  PWM4 : Outport  Port=4
  wires:
  Mux/1 -> Gain/1
  Gain/1 -> Demux/1
  Demux/3 -> PWM3/1
  Demux/1 -> PWM1/1
  Demux/2 -> PWM2/1
  Droll/1 -> Mux/3
  OMEGA/1 -> Mux/1
  Dyaw/1 -> Mux/4
  Dpitch/1 -> Mux/2
  Demux/4 -> PWM4/1

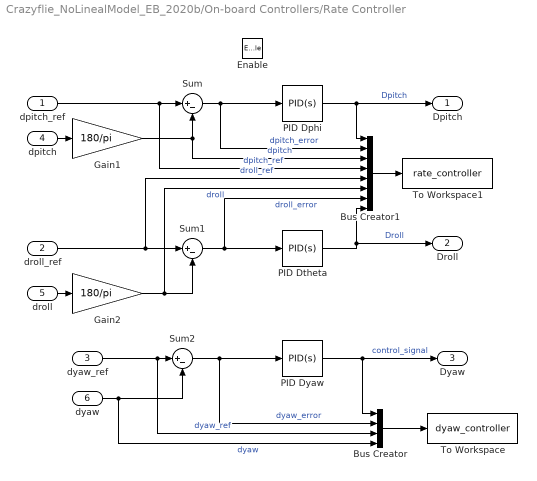
== system Crazyflie_NoLinealModel_EB_2020b/On-board Controllers/Rate Controller ==
  dpitch_ref : Inport
  droll_ref : Inport  Port=2
  dyaw_ref : Inport  Port=3
  dpitch : Inport  Port=4
  droll : Inport  Port=5
  dyaw : Inport  Port=6
  Enable : EnablePort
  Bus Creator : BusCreator  Inputs=4
  Bus Creator1 : BusCreator  Inputs=8
  Gain1 : Gain  Gain=180/pi
  Gain2 : Gain  Gain=180/pi
  PID Dphi : pid_lib/PID Controller  Controller=PID  Form=Parallel  TimeDomain=Continuous-time  UseExternalTs=off  SampleTime=-1  IntegratorMethod=Forward Euler  FilterMethod=Forward Euler  ControllerParametersSource=internal  P=Dphi_s(1)  I=Dphi_s(2)  D=Dphi_s(3)  UseFilter=on  N=100  TunerSelectOption=Transfer Function Based (PID Tuner App)  InitialConditionSource=internal  InitialConditionForIntegrator=0  InitialConditionForFilter=0  DifferentiatorICPrevScaledInput=0  ExternalReset=none  TrackingMode=off  Kt=1  LimitOutput=off  SatLimitsSource=internal  UpperSaturationLimit=inf  LowerSaturationLimit=-inf  LinearizeAsGain=on  AntiWindupMode=none  Kb=1  POutMin=[]  POutMax=[]  IOutMin=[]  IOutMax=[]  DOutMin=[]  DOutMax=[]  NOutMin=[]  NOutMax=[]  SumOutMin=[]  SumOutMax=[]  SaturationOutMin=[]  SaturationOutMax=[]  PParamMin=[]  PParamMax=[]  IParamMin=[]  IParamMax=[]  DParamMin=[]  DParamMax=[]  NParamMin=[]  NParamMax=[]  KbParamMin=[]  KbParamMax=[]  KtParamMin=[]  KtParamMax=[]  KbOutMin=[]  KbOutMax=[]  KtOutMin=[]  KtOutMax=[]  IntegratorOutMin=[]  IntegratorOutMax=[]  FilterOutMin=[]  FilterOutMax=[]  SumI1OutMin=[]  SumI1OutMax=[]  SumI2OutMin=[]  SumI2OutMax=[]  SumI3OutMin=[]  SumI3OutMax=[]  SumI4OutMin=[]  SumI4OutMax=[]  SumDOutMin=[]  SumDOutMax=[]  DifferentiatorOutMin=[]  DifferentiatorOutMax=[]  FilterDiffOutCoefMin=[]  FilterDiffOutCoefMax=[]  ReciprocalOutMin=[]  ReciprocalOutMax=[]  SumDenOutMin=[]  SumDenOutMax=[]  SumNumOutMin=[]  SumNumOutMax=[]  DivideOutMin=[]  DivideOutMax=[]  UdiffTsProdOutMin=[]  UdiffTsProdOutMax=[]  NTsProdOutMin=[]  NTsProdOutMax=[]  UintegralTsProdOutMin=[]  UintegralTsProdOutMax=[]  UngainTsProdOutMin=[]  UngainTsProdOutMax=[]  IntegratorContinuousStateAttributes=''  IntegratorStateMustResolveToSignalObject=off  IntegratorRTWStateStorageClass=Auto  FilterContinuousStateAttributes=''  FilterStateMustResolveToSignalObject=off  FilterRTWStateStorageClass=Auto  ParallelPVariant=InternalParameters  IdealPVariant=Disabled  IVariant=InternalParameters  DVariant=InternalParameters  IntegratorVariant=Continuous  SatVariant=Disabled  AWVariant=Passthrough  PCopyVariant=Disabled  TRVariant=Disabled  FdbkBlocksVariant=Forward  IdealPFdbkVariant=Disabled  SatFdbkVariant=Disabled  DerivativeFilterVariant=ContFilter  NVariant=InternalParameters  NCopyVariant=Disabled  FilterICVariant=InternalICsFilter  IntegratorICVariant=InternalICs  ExternalResetVariant=Disabled  TRSumVariant=Passthrough  SumFdbkVariant=Disabled  SumVariant=Sum_PID  TsampFilterVariant=InternalTs  TsampNgainVariant=Passthrough  TsampIntegralVariant=Passthrough  ExternalSaturationOutDataTypeStr=Inherit: Same as second input
  PID Dtheta : pid_lib/PID Controller  Controller=PID  Form=Parallel  TimeDomain=Continuous-time  UseExternalTs=off  SampleTime=-1  IntegratorMethod=Forward Euler  FilterMethod=Forward Euler  ControllerParametersSource=internal  P=Dtheta_s(1)  I=Dtheta_s(2)  D=Dtheta_s(3)  UseFilter=on  N=100  TunerSelectOption=Transfer Function Based (PID Tuner App)  InitialConditionSource=internal  InitialConditionForIntegrator=0  InitialConditionForFilter=0  DifferentiatorICPrevScaledInput=0  ExternalReset=none  TrackingMode=off  Kt=1  LimitOutput=off  SatLimitsSource=internal  UpperSaturationLimit=inf  LowerSaturationLimit=-inf  LinearizeAsGain=on  AntiWindupMode=none  Kb=1  POutMin=[]  POutMax=[]  IOutMin=[]  IOutMax=[]  DOutMin=[]  DOutMax=[]  NOutMin=[]  NOutMax=[]  SumOutMin=[]  SumOutMax=[]  SaturationOutMin=[]  SaturationOutMax=[]  PParamMin=[]  PParamMax=[]  IParamMin=[]  IParamMax=[]  DParamMin=[]  DParamMax=[]  NParamMin=[]  NParamMax=[]  KbParamMin=[]  KbParamMax=[]  KtParamMin=[]  KtParamMax=[]  KbOutMin=[]  KbOutMax=[]  KtOutMin=[]  KtOutMax=[]  IntegratorOutMin=[]  IntegratorOutMax=[]  FilterOutMin=[]  FilterOutMax=[]  SumI1OutMin=[]  SumI1OutMax=[]  SumI2OutMin=[]  SumI2OutMax=[]  SumI3OutMin=[]  SumI3OutMax=[]  SumI4OutMin=[]  SumI4OutMax=[]  SumDOutMin=[]  SumDOutMax=[]  DifferentiatorOutMin=[]  DifferentiatorOutMax=[]  FilterDiffOutCoefMin=[]  FilterDiffOutCoefMax=[]  ReciprocalOutMin=[]  ReciprocalOutMax=[]  SumDenOutMin=[]  SumDenOutMax=[]  SumNumOutMin=[]  SumNumOutMax=[]  DivideOutMin=[]  DivideOutMax=[]  UdiffTsProdOutMin=[]  UdiffTsProdOutMax=[]  NTsProdOutMin=[]  NTsProdOutMax=[]  UintegralTsProdOutMin=[]  UintegralTsProdOutMax=[]  UngainTsProdOutMin=[]  UngainTsProdOutMax=[]  IntegratorContinuousStateAttributes=''  IntegratorStateMustResolveToSignalObject=off  IntegratorRTWStateStorageClass=Auto  FilterContinuousStateAttributes=''  FilterStateMustResolveToSignalObject=off  FilterRTWStateStorageClass=Auto  ParallelPVariant=InternalParameters  IdealPVariant=Disabled  IVariant=InternalParameters  DVariant=InternalParameters  IntegratorVariant=Continuous  SatVariant=Disabled  AWVariant=Passthrough  PCopyVariant=Disabled  TRVariant=Disabled  FdbkBlocksVariant=Forward  IdealPFdbkVariant=Disabled  SatFdbkVariant=Disabled  DerivativeFilterVariant=ContFilter  NVariant=InternalParameters  NCopyVariant=Disabled  FilterICVariant=InternalICsFilter  IntegratorICVariant=InternalICs  ExternalResetVariant=Disabled  TRSumVariant=Passthrough  SumFdbkVariant=Disabled  SumVariant=Sum_PID  TsampFilterVariant=InternalTs  TsampNgainVariant=Passthrough  TsampIntegralVariant=Passthrough  ExternalSaturationOutDataTypeStr=Inherit: Same as second input
  PID Dyaw : pid_lib/PID Controller  Controller=PID  Form=Parallel  TimeDomain=Continuous-time  UseExternalTs=off  SampleTime=-1  IntegratorMethod=Forward Euler  FilterMethod=Forward Euler  ControllerParametersSource=internal  P=Dpsi_s(1)  I=Dpsi_s(2)  D=Dpsi_s(3)  UseFilter=on  N=100  TunerSelectOption=Transfer Function Based (PID Tuner App)  InitialConditionSource=internal  InitialConditionForIntegrator=0  InitialConditionForFilter=0  DifferentiatorICPrevScaledInput=0  ExternalReset=none  TrackingMode=off  Kt=1  LimitOutput=off  SatLimitsSource=internal  UpperSaturationLimit=inf  LowerSaturationLimit=-inf  LinearizeAsGain=on  AntiWindupMode=none  Kb=1  POutMin=[]  POutMax=[]  IOutMin=[]  IOutMax=[]  DOutMin=[]  DOutMax=[]  NOutMin=[]  NOutMax=[]  SumOutMin=[]  SumOutMax=[]  SaturationOutMin=[]  SaturationOutMax=[]  PParamMin=[]  PParamMax=[]  IParamMin=[]  IParamMax=[]  DParamMin=[]  DParamMax=[]  NParamMin=[]  NParamMax=[]  KbParamMin=[]  KbParamMax=[]  KtParamMin=[]  KtParamMax=[]  KbOutMin=[]  KbOutMax=[]  KtOutMin=[]  KtOutMax=[]  IntegratorOutMin=[]  IntegratorOutMax=[]  FilterOutMin=[]  FilterOutMax=[]  SumI1OutMin=[]  SumI1OutMax=[]  SumI2OutMin=[]  SumI2OutMax=[]  SumI3OutMin=[]  SumI3OutMax=[]  SumI4OutMin=[]  SumI4OutMax=[]  SumDOutMin=[]  SumDOutMax=[]  DifferentiatorOutMin=[]  DifferentiatorOutMax=[]  FilterDiffOutCoefMin=[]  FilterDiffOutCoefMax=[]  ReciprocalOutMin=[]  ReciprocalOutMax=[]  SumDenOutMin=[]  SumDenOutMax=[]  SumNumOutMin=[]  SumNumOutMax=[]  DivideOutMin=[]  DivideOutMax=[]  UdiffTsProdOutMin=[]  UdiffTsProdOutMax=[]  NTsProdOutMin=[]  NTsProdOutMax=[]  UintegralTsProdOutMin=[]  UintegralTsProdOutMax=[]  UngainTsProdOutMin=[]  UngainTsProdOutMax=[]  IntegratorContinuousStateAttributes=''  IntegratorStateMustResolveToSignalObject=off  IntegratorRTWStateStorageClass=Auto  FilterContinuousStateAttributes=''  FilterStateMustResolveToSignalObject=off  FilterRTWStateStorageClass=Auto  ParallelPVariant=InternalParameters  IdealPVariant=Disabled  IVariant=InternalParameters  DVariant=InternalParameters  IntegratorVariant=Continuous  SatVariant=Disabled  AWVariant=Passthrough  PCopyVariant=Disabled  TRVariant=Disabled  FdbkBlocksVariant=Forward  IdealPFdbkVariant=Disabled  SatFdbkVariant=Disabled  DerivativeFilterVariant=ContFilter  NVariant=InternalParameters  NCopyVariant=Disabled  FilterICVariant=InternalICsFilter  IntegratorICVariant=InternalICs  ExternalResetVariant=Disabled  TRSumVariant=Passthrough  SumFdbkVariant=Disabled  SumVariant=Sum_PID  TsampFilterVariant=InternalTs  TsampNgainVariant=Passthrough  TsampIntegralVariant=Passthrough  ExternalSaturationOutDataTypeStr=Inherit: Same as second input
  Sum : Sum  Inputs=|+-
  Sum1 : Sum  Inputs=|+-
  Sum2 : Sum  Inputs=|+-
  To Workspace : ToWorkspace  VariableName=dyaw_controller  SaveFormat=Timeseries  SampleTime=-1
  To Workspace1 : ToWorkspace  VariableName=rate_controller  SaveFormat=Timeseries  SampleTime=-1
  Dpitch : Outport
  Droll : Outport  Port=2
  Dyaw : Outport  Port=3
  wires:
  dyaw/1 -> Bus Creator/4, Sum2/2  "dyaw"
  Sum/1 -> PID Dphi/1, Bus Creator1/2  "dpitch_error"
  Bus Creator1/1 -> To Workspace1/1
  dpitch/1 -> Gain1/1
  droll/1 -> Gain2/1
  PID Dyaw/1 -> Bus Creator/1, Dyaw/1  "control_signal"
  Gain1/1 -> Bus Creator1/3, Sum/2  "dpitch"
  Gain2/1 -> Bus Creator1/6, Sum1/2  "droll"
  droll_ref/1 -> Bus Creator1/5, Sum1/1  "droll_ref"
  dyaw_ref/1 -> Bus Creator/3, Sum2/1  "dyaw_ref"
  dpitch_ref/1 -> Bus Creator1/4, Sum/1  "dpitch_ref"
  PID Dphi/1 -> Dpitch/1, Bus Creator1/1  "Dpitch"
  Sum1/1 -> PID Dtheta/1, Bus Creator1/7  "droll_error"
  Bus Creator/1 -> To Workspace/1
  Sum2/1 -> PID Dyaw/1, Bus Creator/2  "dyaw_error"
  PID Dtheta/1 -> Bus Creator1/8, Droll/1  "Droll"

== system Crazyflie_NoLinealModel_EB_2020b/Event Trigered/Subsystem3/If Action Subsystem4 ==
  In2 : Inport
  Enable : EnablePort
  Out2 : Outport
  wires:
  In2/1 -> Out2/1

== system Crazyflie_NoLinealModel_EB_2020b/Event Trigered/Subsystem4/If Action Subsystem4 ==
  In2 : Inport
  Enable : EnablePort
  Out2 : Outport
  wires:
  In2/1 -> Out2/1

== matlab function Crazyflie_NoLinealModel_EB_2020b/Crazyflie2.0  Non-Linear Model/MATLAB Function ==
  data: uvw input; xyz_dot output; angles input
function xyz_dot  = Position(uvw,angles)
xyz_dot = zeros(3,1);
phi = angles(1); %*pi/180;
theta = angles(2); %*pi/180;
psi = angles(3); %*pi/180;
Tb_o = [cos(theta)*cos(psi)                                cos(theta)*sin(psi)                             -sin(theta)  ;   %BBF > Inertial rotation matrix
        sin(phi)*sin(theta)*cos(psi)-cos(phi)*sin(psi)    sin(phi)*sin(theta)*sin(psi)+cos(phi)*cos(psi)  sin(phi)*cos(theta) ;
        cos(phi)*sin(theta)*cos(psi)+sin(phi)*sin(psi)    cos(phi)*sin(theta)*sin(psi)-sin(phi)*cos(psi)   cos(phi)*cos(theta)];

xyz_dot = (Tb_o')*uvw;
end

== matlab function Crazyflie_NoLinealModel_EB_2020b/Off-board Controllers [100Hz]/Triggered Subsystem2/Error to Body Frame ==
  data: xc input; xbe output; yc input; x input; y input; psi input; ybe output
function [xbe, ybe] = fcn(xc, yc, x, y, psi)

xe = xc-x;
ye = yc-y;

xbe = xe*cos(psi)+ye*sin(psi);
ybe = -xe*sin(psi)+ye*cos(psi);

== matlab function Crazyflie_NoLinealModel_EB_2020b/Crazyflie2.0  Non-Linear Model/MATLAB Function1 ==
  data: pqr input; angles_dot output; angles input
function angles_dot  = Angle(pqr,angles)
angles_dot = zeros(3,1);
phi = angles(1); %*pi/180;
theta = angles(2); %*pi/180;

H = [1    sin(phi)*tan(theta)     cos(phi)*tan(theta)
     0       cos(phi)                 -sin(phi)   
     0       sin(phi)/cos(theta)    cos(phi)/cos(theta)];
angles_dot = H*pqr;
end

== matlab function Crazyflie_NoLinealModel_EB_2020b/Event Trigered/Z Trigger Code ==
  settings: updateMethod=DISCRETE  sampleTime=0.001
  data: Time input; Z_enable output boolean; ref input; dron input; threshold input; lastZSampleTime data_store_memory; lastZValue data_store_memory; Event_signal output; Self_signal output; period input
function [Z_enable, Event_signal, Self_signal] = fcn(Time, ref, dron, threshold, period)
%#codegen
global lastZSampleTime;
global lastZValue;

signal = abs(dron - lastZValue);
error = ref - dron;
t_signal = Time - lastZSampleTime;
u = false;
Event_signal = false;
Self_signal = false;
% Condición cota
if(signal >= threshold || Time == 0)
   u = true;
   Event_signal = true;
   lastZValue = dron;
   lastZSampleTime = Time;
end

% Condición temporal
if(t_signal>=period)
    u = true;
    Self_signal = true;
    lastZValue = dron;
    lastZSampleTime = Time;
end

% % Condición error
% if(t_signal>=0.05 && z_error>0.1)
%     u = true;
%     lastZValue = Z_dron;
%     lastZSampleTime = Time;
% end
Z_enable = u;

== matlab function Crazyflie_NoLinealModel_EB_2020b/Crazyflie2.0  Non-Linear Model/MATLAB Function2 ==
  data: uvw input; uvw_dot output; pqr input; angles input; F input
function uvw_dot  = Forces(uvw,pqr,angles,F)
uvw_dot = zeros(3,1);
Force = [0;0;F];
g_o = [0;0;-9.81];
phi = angles(1); %*pi/180;
theta = angles(2); %*pi/180;
psi = angles(3); %*pi/180;
Rx = [1 0 0; 0 cos(phi) sin(phi); 0 -sin(phi) cos(phi)];
Ry = [cos(theta) 0 -sin(theta); 0 1 0; sin(theta) 0 cos(theta)];
Rz = [cos(psi) sin(psi) 0; -sin(psi) cos(psi) 0; 0 0 1];
Tb_o = Rx*Ry*Rz;
% Tb_o = [cos(theta)*cos(psi)                                cos(theta)*sin(psi)                             -sin(theta)  ;   %BBF > Inertial rotation matrix
%         sin(phi)*sin(theta)*cos(psi)-cos(phi)*sin(psi)    sin(phi)*sin(theta)*sin(psi)+cos(phi)*cos(psi)  sin(phi)*cos(theta) ;
%         cos(phi)*sin(theta)*cos(psi)+sin(phi)*sin(psi)    cos(phi)*sin(theta)*sin(psi)-sin(phi)*cos(psi)   cos(phi)*cos(theta)];

    uvw_dot = Force + Tb_o*g_o - cross(pqr,uvw);

end

== matlab function Crazyflie_NoLinealModel_EB_2020b/Crazyflie2.0  Non-Linear Model/MATLAB Function3 ==
  data: pqr_dot output; pqr input; M input
function pqr_dot  = Moments(pqr,M)
pqr_dot = zeros(3,1);
Ixx =  1.395e-05;  %2.3951e-5; %1.39e-05; %2.51943e-5; % % %
Iyy = 1.436e-05; %2.3951e-5; %1.436e-05; % 2.54379e-5; % %         %
Izz =  2.173e-05;  %3.2347e-5; %2.173e-05 ; %4.51407e-5; % %         %;%0.160;
J = diag([Ixx Iyy Izz]);    %   I  Flyer rotational inertia matrix     3x3
pqr_dot = inv(J)*(M-cross(pqr,J*pqr));
end

== matlab function Crazyflie_NoLinealModel_EB_2020b/Event Trigered/XY Trigger Code ==
  settings: updateMethod=DISCRETE  sampleTime=0.001
  data: Time input; XY_enable output boolean; xref input; yref input; xdron input; ydron input; threshold input; Event_signal output; Self_signal output; period input; lastXYSampleTime data_store_memory; lastXValue data_store_memory; lastYValue data_store_memory
function [XY_enable, Event_signal, Self_signal] = fcn(Time, xref, yref, xdron, ydron, threshold, period)
%#codegen
global lastXYSampleTime;
global lastXValue;
global lastYValue;

xerror = xref - xdron;
yerror = yref - ydron;
xysignal = abs(sqrt(xdron^2+ydron^2)-sqrt(lastXValue^2+lastYValue^2));
t_signal = Time - lastXYSampleTime;
u = false;
Event_signal = false;
Self_signal = false;

% Condición cota
if(xysignal >= threshold || Time == 0)
   u = true;
   Event_signal = true;
   lastXValue = xdron;
   lastYValue = ydron;
   lastXYSampleTime = Time;
end

% Condición temporal
if(t_signal>=period)
   u = true;
   Self_signal = true;
   lastXValue = xdron;
   lastYValue = ydron;
   lastXYSampleTime = Time;
end

% % Condición error
% if(t_signal>=0.05 && z_error>0.1)
%     u = true;
%     lastZValue = Z_dron;
%     lastZSampleTime = Time;
% end
XY_enable = u;

== matlab function Crazyflie_NoLinealModel_EB_2020b/Event Trigered/Yaw Trigger Code ==
  settings: updateMethod=DISCRETE  sampleTime=0.001
  data: Time input; Yaw_enable output boolean; ref input; dron input; threshold input; lastYawSampleTime data_store_memory; lastYawValue data_store_memory; Event_signal output; Self_signal output; period input
function [Yaw_enable, Event_signal, Self_signal] = fcn(Time, ref, dron, threshold, period)
%#codegen
global lastYawSampleTime;
global lastYawValue;

signal = abs(dron - lastYawValue);
error = ref - dron;
t_signal = Time - lastYawSampleTime;
u = false;
Event_signal = false;
Self_signal = false;
% Condición cota
if(signal >= threshold || Time == 0)
   u = true;
   Event_signal = true;
   lastYawValue = dron;
   lastYawSampleTime = Time;
end

% Condición temporal
if(t_signal>=period)
    u = true;
    Self_signal = true;
    lastYawValue = dron;
    lastYawSampleTime = Time;
end

Yaw_enable = u;
